simulink model "test_discrete_ss_tv_model"  (R2020a)
settings: Solver=FixedStepDiscrete  StartTime=0.0  StopTime=t(end)  FixedStep=1  RelTol=1e-3
values from neighbouring files (symbols this model uses):
  A0 = T*A0*inv(T)    [test_continuous_ss_lpv.m]    (also in test_continuous_ss_tv.m; test_discrete_ss_lpv.m; test_discrete_ss_tv.m)
  A1 = 1e-10*round(2*(rand(n,n)-0.5))    [test_continuous_ss_lpv.m]    (also in test_continuous_ss_tv.m; test_discrete_ss_lpv.m; test_discrete_ss_tv.m)
  B0 = rand(n,m)    [test_continuous_ss_lpv.m]    (also in test_continuous_ss_tv.m; test_discrete_ss_lpv.m; test_discrete_ss_tv.m)
  B1 = 1e-3*round(2*(rand(n,m)-0.5))    [test_continuous_ss_lpv.m]    (also in test_continuous_ss_tv.m = round(2*(rand(n,m)-0.5)); test_discrete_ss_lpv.m; test_discrete_ss_tv.m = round(2*(rand(n,m)-0.5)))
  C0 = rand(p,n)    [test_continuous_ss_lpv.m]    (also in test_continuous_ss_tv.m; test_discrete_ss_lpv.m; test_discrete_ss_tv.m)
  C1 = 1e-3*round(2*(rand(p,n)-0.5))    [test_continuous_ss_lpv.m]    (also in test_continuous_ss_tv.m = round(2*(rand(p,n)-0.5)); test_discrete_ss_lpv.m; test_discrete_ss_tv.m = round(2*(rand(p,n)-0.5)))
  D0 = rand(p,m)    [test_continuous_ss_lpv.m]    (also in test_continuous_ss_tv.m; test_discrete_ss_lpv.m; test_discrete_ss_tv.m)
  D1 = 1e-3*round(2*(rand(p,m)-0.5))    [test_continuous_ss_lpv.m]    (also in test_continuous_ss_tv.m = round(2*(rand(p,m)-0.5)); test_discrete_ss_lpv.m; test_discrete_ss_tv.m = round(2*(rand(p,m)-0.5)))
  initial_state = rand(n,1)    [test_continuous_ss_lpv.m]    (also in test_continuous_ss_ti.m; test_continuous_ss_tv.m; test_discrete_ss_lpv.m; test_discrete_ss_ti.m)
settings Model: Creator=bascetta  LastModifiedBy=bascetta

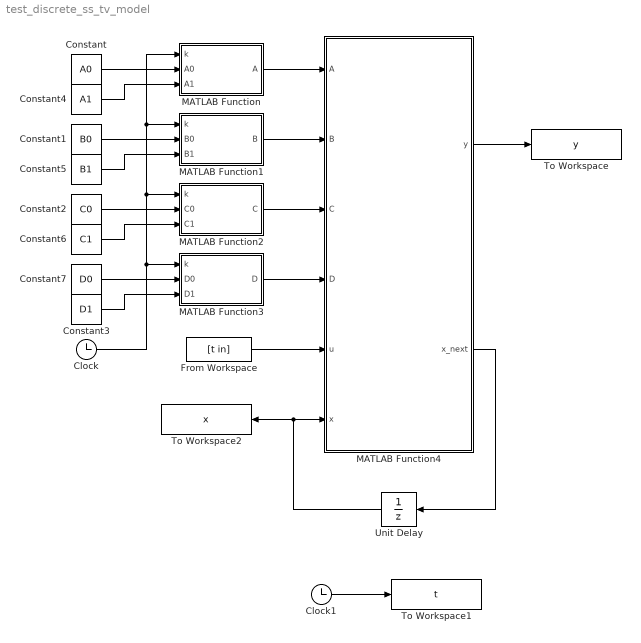
== system test_discrete_ss_tv_model ==
  Clock : Clock
  Clock1 : Clock
  Constant : Constant  Value=A0  VectorParams1D=off
  Constant1 : Constant  Value=B0  VectorParams1D=off
  Constant2 : Constant  Value=C0  VectorParams1D=off
  Constant3 : Constant  Value=D1  VectorParams1D=off
  Constant4 : Constant  Value=A1  VectorParams1D=off
  Constant5 : Constant  Value=B1  VectorParams1D=off
  Constant6 : Constant  Value=C1  VectorParams1D=off
  Constant7 : Constant  Value=D0  VectorParams1D=off
  From Workspace : FromWorkspace  VariableName=[t in]  SampleTime=1
  MATLAB Function : MATLAB Function  TreatAsAtomicUnit=on
  MATLAB Function1 : MATLAB Function  TreatAsAtomicUnit=on
  MATLAB Function2 : MATLAB Function  TreatAsAtomicUnit=on
  MATLAB Function3 : MATLAB Function  TreatAsAtomicUnit=on
  MATLAB Function4 : MATLAB Function  TreatAsAtomicUnit=on
  To Workspace : ToWorkspace  VariableName=y  SampleTime=-1
      settings: Save2DSignal=2-D array (concatenate along first dimension)
  To Workspace1 : ToWorkspace  VariableName=t  SampleTime=-1
      settings: Save2DSignal=2-D array (concatenate along first dimension)
  To Workspace2 : ToWorkspace  VariableName=x  SampleTime=-1
      settings: Save2DSignal=2-D array (concatenate along first dimension)
  Unit Delay : UnitDelay  InitialCondition=initial_state  SampleTime=-1  HasFrameUpgradeWarning=on
  wires:
  From Workspace/1 -> MATLAB Function4/5(u)
  MATLAB Function4/1(y) -> To Workspace/1
  Clock/1 -> MATLAB Function/1(k), MATLAB Function1/1(k), MATLAB Function2/1(k), MATLAB Function3/1(k)
  MATLAB Function/1(A) -> MATLAB Function4/1(A)
  MATLAB Function1/1(B) -> MATLAB Function4/2(B)
  MATLAB Function2/1(C) -> MATLAB Function4/3(C)
  MATLAB Function3/1(D) -> MATLAB Function4/4(D)
  MATLAB Function4/2(x_next) -> Unit Delay/1
  Unit Delay/1 -> To Workspace2/1, MATLAB Function4/6(x)
  Clock1/1 -> To Workspace1/1
  Constant/1 -> MATLAB Function/2(A0)
  Constant4/1 -> MATLAB Function/3(A1)
  Constant1/1 -> MATLAB Function1/2(B0)
  Constant5/1 -> MATLAB Function1/3(B1)
  Constant2/1 -> MATLAB Function2/2(C0)
  Constant6/1 -> MATLAB Function2/3(C1)
  Constant7/1 -> MATLAB Function3/2(D0)
  Constant3/1 -> MATLAB Function3/3(D1)

== matlab function test_discrete_ss_tv_model/MATLAB Function1 ==
  data: k input; B output; B0 input; B1 input
function B = B_matrix(k,B0,B1)

B = B0+B1*k^0.5;

== matlab function test_discrete_ss_tv_model/MATLAB Function ==
  data: k input; A output; A0 input; A1 input
function A = A_matrix(k,A0,A1)

A = A0+A1*k^0.5;

== matlab function test_discrete_ss_tv_model/MATLAB Function2 ==
  data: k input; C output; C0 input; C1 input
function C = C_matrix(k,C0,C1)

C = C0+C1*k^0.5;

== matlab function test_discrete_ss_tv_model/MATLAB Function3 ==
  data: k input; D output; D0 input; D1 input
function D = D_matrix(k,D0,D1)

D = D0+D1*k^0.5;

== matlab function test_discrete_ss_tv_model/MATLAB Function4 ==
  data: A input; B input; C input; D input; u input; x input; y output; x_next output
function [y,x_next] = statespace_model(A,B,C,D,u,x)

x_next = zeros(size(A,1),1);
y = zeros(size(C,1),1);

x_next = A*x+B*u;
y      = C*x+D*u;
